simulink model "FOC"  (R2020b)
settings: Solver=ode45  StartTime=0.0  StopTime=1  MaxStep=1e-6  RelTol=1e-3
undefined symbols (not defined in the file): AlphaQ15, CurKiQ9, CurKpQ9, CurMax, CurTs, F, J, Ls, Mode, Np, Rs, SpdKiQ11, SpdKpQ11, TargetId, TargetIq, TargetSpd, TargetUd, TargetUq, Tf, Tn, Udc, VolMax, wn
libraries: powerlib x5, powerlib_meascontrol x1, simulink x1
settings Model: SimulationMode=accelerator  Creator=LFL  LastModifiedBy=Administrator
settings DataIOCC: ReturnWorkspaceOutputs=off
settings DebuggingCC: ArithmeticOperatorsInVariantConditions=warning
settings SFSimCC: SimUseLocalCustomCode=off  CustomCodeUndefinedFunction=UseInterfaceOnly
settings RTWCC: RTWUseLocalCustomCode=off

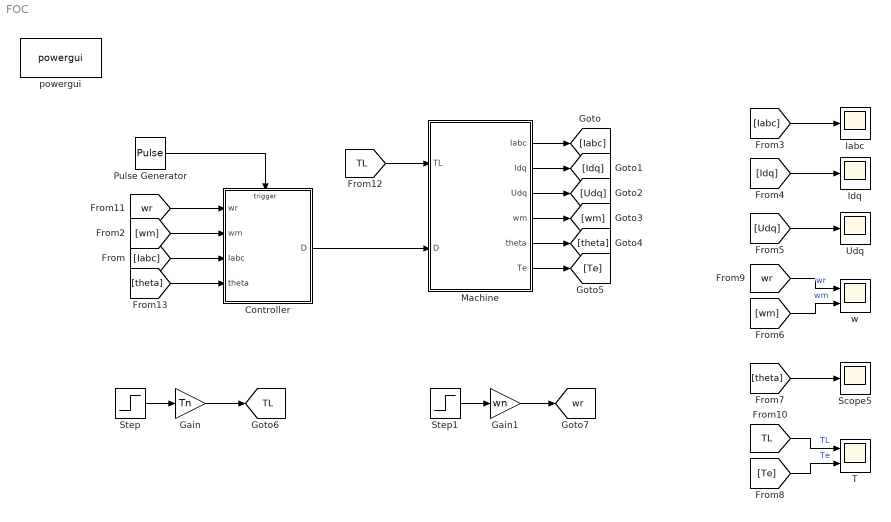
== system FOC ==
  Controller : Subsystem  TreatAsAtomicUnit=on
  Gain : Gain  Gain=Tn
  Gain1 : Gain  Gain=wn
  Iabc : Scope
  Idq : Scope
  Machine : Subsystem
  Pulse Generator : DiscretePulseGenerator  PulseType=Time based  Period=CurTs  PulseWidth=50
  Scope5 : Scope
  Step : Step  Time=0.1  SampleTime=0
  Step1 : Step  Time=0  SampleTime=0
  T : Scope  NumInputPorts=2
  Udq : Scope
  powergui : powerlib/powergui  Priority=1  SimulationMode=Discrete  SampleTime=1e-6  frequency=60  Iterations=50  frequencyindice=0  Pbase=100e6  ErrMax=1e-4  UnitsV=kV  UnitsW=MW  buscounter=0  FunctionMessages=off  echomessages=off  EnableUseOfTLC=off  CurrentSourceSwitches=off  DisableSnubberDevices=off  DisableRonSwitches=off  DisableVfSwitches=off  DisplayEquations=off  AutomaticDiscreteSolvers=off  SolverType=Tustin/Backward Euler (TBE)  Interpol=off  ExternalGateDelay=off  methode=off  Ts=100  x0status=blocks  SPID=on  SwTol=0  HookPort=off  NonlinearTolerance=1e-4  nMaxIteration=100  ContinueOnMaxIteration=off  RestoreLinks=warning  ResistiveCurrentMeasurement=off  Frange=[0:2:500]  Ylog=off  Xlog=on  ShowGrid=off  save=off  variable=ZData  structure=0  ZoomFFT=off  StartTime=0.0  cycles=1  DisplayStyle=1  fundamental=60  FreqAxis=off  MaxFrequency=1000  frequencyindicesteady=1  RmsSteady=1  display=off
  w : Scope  NumInputPorts=2
  tag scope: TL=global, wr=global
  wires:
  Pulse Generator/1 -> Controller/Trigger
  Machine/1(Iabc) -> [Iabc]
  Machine/2(Idq) -> [Idq]
  Machine/3(Udq) -> [Udq]
  Machine/4(wm) -> [wm]
  Machine/5(theta) -> [theta]
  Machine/6(Te) -> [Te]
  [Iabc] -> Controller/3(Iabc)
  [wm] -> Controller/2(wm)
  [Iabc] -> Iabc/1
  [Udq] -> Udq/1
  [wm] -> w/2  "wm"
  [wr] -> w/1  "wr"
  [TL] -> T/1  "TL"
  [Te] -> T/2  "Te"
  [theta] -> Scope5/1
  [Idq] -> Idq/1
  [wr] -> Controller/1(wr)
  [TL] -> Machine/1(TL)
  [theta] -> Controller/4(theta)
  Step/1 -> Gain/1
  Gain/1 -> [TL]
  Step1/1 -> Gain1/1
  Gain1/1 -> [wr]
  Controller/1(D) -> Machine/2(D)

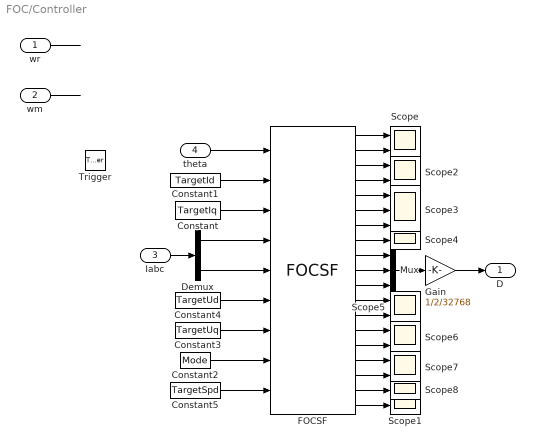
== system FOC/Controller ==
  wr : Inport
  wm : Inport  Port=2
  Iabc : Inport  Port=3
  theta : Inport  Port=4
  Trigger : TriggerPort  VariantControl=Variant
  Constant : Constant  Value=TargetIq
  Constant1 : Constant  Value=TargetId
  Constant2 : Constant  Value=Mode
  Constant3 : Constant  Value=TargetUq
  Constant4 : Constant  Value=TargetUd
  Constant5 : Constant  Value=TargetSpd
  Demux : Demux  Outputs=3
  FOCSF : S-Function  FunctionName=FOCSF  Parameters=Np CurKp CurKi VolMax SpdKp SpdKi CurMax Alpha  SFunctionDeploymentMode=off  EnableBusSupport=off  mask{Np=Np, CurKp=CurKpQ9, CurKi=CurKiQ9, VolMax=VolMax, SpdKp=SpdKpQ11, SpdKi=SpdKiQ11, CurMax=CurMax, Alpha=AlphaQ15}
      mask Display:
      | port_label('input',  1,  'Theta')
      | port_label('input',  2,  'TargetId')
      | port_label('input',  3,  'TargetIq')
      | port_label('input',  4,  'Ia')
      | port_label('input',  5,  'Ic')
      | port_label('input',  6,  'TargetUd')
      | port_label('input',  7,  'TargetUq')
      | port_label('input',  8,  'Mode')
      | port_label('output', 1,  'SinTheta')
      | port_label('output', 2,  'CosTheta')
      | port_label('output', 3,  'Ux')
      | port_label('output', 4,  'Uy')
      | port_label('output', 5,  'U1')
      | port_label('output', 6,  'U2')
      | port_label('output', 7,  'U3')
      | port_label('output', 8,  'Sector')
      | port_label('output', 9,  'CCRa')
      | port_label('output', 10, 'CCRb')
      | port_label('output', 11, 'CCRc')
      | port_label('output', 12, 'Ix')
      | port_label('output', 13, 'Iy')
      | port_label('output', 14, 'PresentId')
      | port_label('output', 15, 'PresentIq')
      | port_label('output', 16, 'PresentUd')
      | port_label('output', 17, 'PresentUq')
      | port_label('output', 18, 'PresentSpd')
  Gain : Gain  Gain=1/2/32768
  Mux : Mux  Inputs=3
  Scope{,2,5..7} (5 alike) : Scope  NumInputPorts=2
  Scope1 : Scope
  Scope3 : Scope  NumInputPorts=3
  Scope4 : Scope
  Scope8 : Scope
  D : Outport  VectorParamsAs1DForOutWhenUnconnected=off
  wires:
  wr/1 -> ?
  wm/1 -> ?
  theta/1 -> FOCSF/1
  FOCSF/1 -> Scope/1
  FOCSF/2 -> Scope/2
  Constant/1 -> FOCSF/3
  Constant1/1 -> FOCSF/2
  FOCSF/3 -> Scope2/1
  FOCSF/4 -> Scope2/2
  FOCSF/5 -> Scope3/1
  FOCSF/6 -> Scope3/2
  FOCSF/7 -> Scope3/3
  FOCSF/8 -> Scope4/1
  FOCSF/9 -> Mux/1
  FOCSF/10 -> Mux/2
  FOCSF/11 -> Mux/3
  Mux/1 -> Gain/1
  Gain/1 -> D/1
  Iabc/1 -> Demux/1
  Demux/1 -> FOCSF/4
  Demux/3 -> FOCSF/5
  FOCSF/13 -> Scope5/2
  FOCSF/12 -> Scope5/1
  FOCSF/14 -> Scope6/1
  FOCSF/15 -> Scope6/2
  FOCSF/16 -> Scope7/1
  FOCSF/17 -> Scope7/2
  FOCSF/18 -> Scope8/1
  Constant2/1 -> FOCSF/8
  Constant3/1 -> FOCSF/7
  Constant4/1 -> FOCSF/6
  Constant5/1 -> FOCSF/9
  FOCSF/19 -> Scope1/1

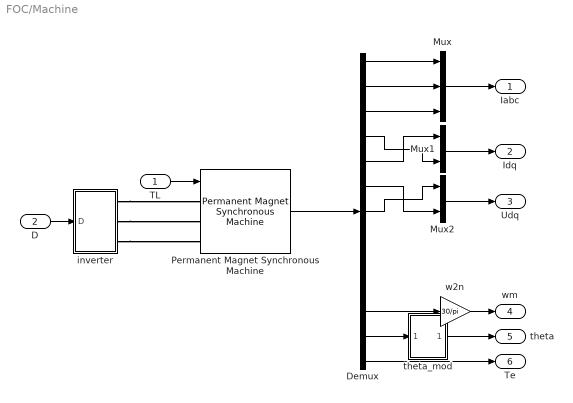
== system FOC/Machine ==
  TL : Inport
  D : Inport  Port=2
  Demux : Demux  Outputs=13
  Mux : Mux  Inputs=3
  Mux1 : Mux  Inputs=2
  Mux2 : Mux  Inputs=2
  Permanent Magnet Synchronous Machine : powerlib/Machines/Permanent Magnet Synchronous Machine  NbPhases=3  FluxDistribution=Sinusoidal  RotorType=Salient-pole  MechanicalLoad=Torque Tm  PresetModel=No  ShowDetailedParameters=on  MeasurementBus=off  Resistance=Rs  Inductance=8.5e-3  dqInductances=[Ls,Ls]  La=0.000395  MachineConstant=Torque Constant (N.m / A_peak)  Flux=0.014667  VoltageCst=13.3012  TorqueCst=Kt  Flat=120  Mechanical=[J F Np Tf]  PolePairs=4  InitialConditions=[0,0, 0,0]  InitialConditions5ph=[0 0 0 0 0 0]  RefAngle=Aligned with phase A axis (original Park)  IterativeDiscreteModel=Trapezoidal non iterative  TsBlock=-1  TsPowergui=0
  inverter : Subsystem
  theta_mod : Subsystem
  w2n : Gain  Gain=30/pi
  Iabc : Outport  VectorParamsAs1DForOutWhenUnconnected=off
  Idq : Outport  Port=2  VectorParamsAs1DForOutWhenUnconnected=off
  Udq : Outport  Port=3  VectorParamsAs1DForOutWhenUnconnected=off
  wm : Outport  Port=4  VectorParamsAs1DForOutWhenUnconnected=off
  theta : Outport  Port=5  VectorParamsAs1DForOutWhenUnconnected=off
  Te : Outport  Port=6  VectorParamsAs1DForOutWhenUnconnected=off
  wires:
  Permanent Magnet Synchronous Machine/1 -> Demux/1
  Demux/1 -> Mux/1
  Demux/2 -> Mux/2
  Demux/3 -> Mux/3
  Mux/1 -> Iabc/1
  Mux1/1 -> Idq/1
  Mux2/1 -> Udq/1
  Demux/11 -> w2n/1
  Demux/12 -> theta_mod/1(In1)
  Demux/13 -> Te/1
  TL/1 -> Permanent Magnet Synchronous Machine/1
  Demux/5 -> Mux1/1
  Demux/4 -> Mux1/2
  Demux/6 -> Mux2/2
  Demux/7 -> Mux2/1
  theta_mod/1(Out1) -> theta/1
  w2n/1 -> wm/1
  D/1 -> inverter/1(D)
  connections:
  inverter/RConn1 -- Permanent Magnet Synchronous Machine/LConn1
  inverter/RConn2 -- Permanent Magnet Synchronous Machine/LConn2
  inverter/RConn3 -- Permanent Magnet Synchronous Machine/LConn3

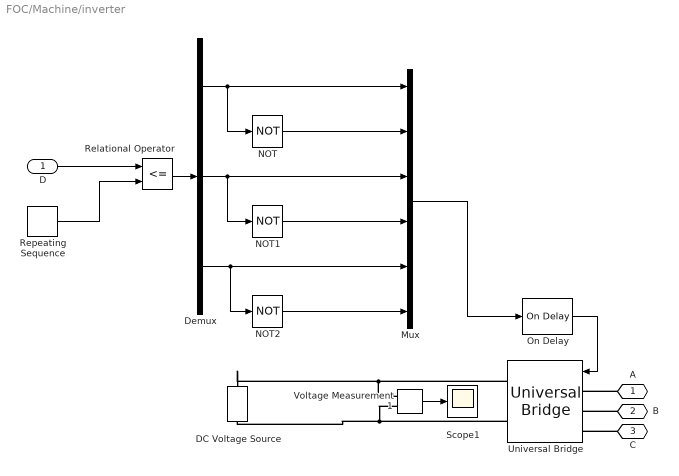
== system FOC/Machine/inverter ==
  D : Inport
  DC Voltage Source : powerlib/Electrical Sources/DC Voltage Source  Amplitude=Udc  Measurements=None
  Demux : Demux  Outputs=3
  Mux : Mux  Inputs=6
  NOT : Logic  Operator=NOT  IconShape=distinctive  AllPortsSameDT=off  OutDataTypeStr=boolean
  NOT1 : Logic  Operator=NOT  IconShape=distinctive  AllPortsSameDT=off  OutDataTypeStr=boolean
  NOT2 : Logic  Operator=NOT  IconShape=distinctive  AllPortsSameDT=off  OutDataTypeStr=boolean
  On Delay : powerlib_meascontrol/Logic/On Delay  DelayType=On delay  delay=Deadtime  ic=0  Ts=0
  Relational Operator : RelationalOperator  Operator=<=  OutDataTypeStr=boolean  RndMeth=Simplest
  Repeating Sequence : simulink/Sources/Repeating Sequence  rep_seq_t=[0 CurTs/2 CurTs]  rep_seq_y=[0 1 0]
  Scope1 : Scope
  Universal Bridge : powerlib/Power Electronics/Universal Bridge  Arms=3  SnubberResistance=1e5  SnubberCapacitance=inf  Device=MOSFET / Diodes  Ron=1e-3  Lon=0  ForwardVoltages="[  0  0  ]"  ForwardVoltage=0  GTOparameters=[ 10e-6 , 20e-6 ]  IGBTparameters=[ 1e-6 , 2e-6 ]  Measurements=None  Measurements_2=None  converterType=Rectifier
  Voltage Measurement1 : powerlib/Measurements/Voltage Measurement  PhasorSimulation=off  OutputType=Complex  PSBequivalent=0
  A : PMIOPort  Side=Right
  B : PMIOPort  Port=2  Side=Right
  C : PMIOPort  Port=3  Side=Right
  wires:
  On Delay/1 -> Universal Bridge/1
  NOT1/1 -> Mux/4
  NOT/1 -> Mux/2
  Demux/1 -> Mux/1, NOT/1
  Demux/3 -> NOT2/1, Mux/5
  Demux/2 -> NOT1/1, Mux/3
  NOT2/1 -> Mux/6
  Relational Operator/1 -> Demux/1
  D/1 -> Relational Operator/1
  Mux/1 -> On Delay/1
  Repeating Sequence/1 -> Relational Operator/2
  Voltage Measurement1/1 -> Scope1/1
  connections:
  A/RConn1 -- Universal Bridge/LConn1
  B/RConn1 -- Universal Bridge/LConn2
  C/RConn1 -- Universal Bridge/LConn3
  DC Voltage Source/RConn1 -- Universal Bridge/RConn1 -- Voltage Measurement1/LConn1
  Voltage Measurement1/LConn2 -- DC Voltage Source/LConn1 -- Universal Bridge/RConn2

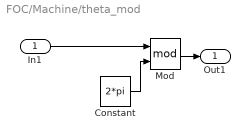
== system FOC/Machine/theta_mod ==
  In1 : Inport
  Constant : Constant  Value=2*pi
  Mod : Math  Operator=mod  SignedPower=on  SaturateOnIntegerOverflow=on
  Out1 : Outport  VectorParamsAs1DForOutWhenUnconnected=off
  wires:
  Mod/1 -> Out1/1
  Constant/1 -> Mod/2
  In1/1 -> Mod/1
